simulink model "laguerre"  (R2018b)
settings: Solver=VariableStepAuto  StartTime=0.0  StopTime=5  RelTol=1e-3
undefined symbols (not defined in the file or in its folder): O, p, sigbuilder_block, sigma, Ts
settings Model: Creator=lenovo  LastModifiedBy=lenovo

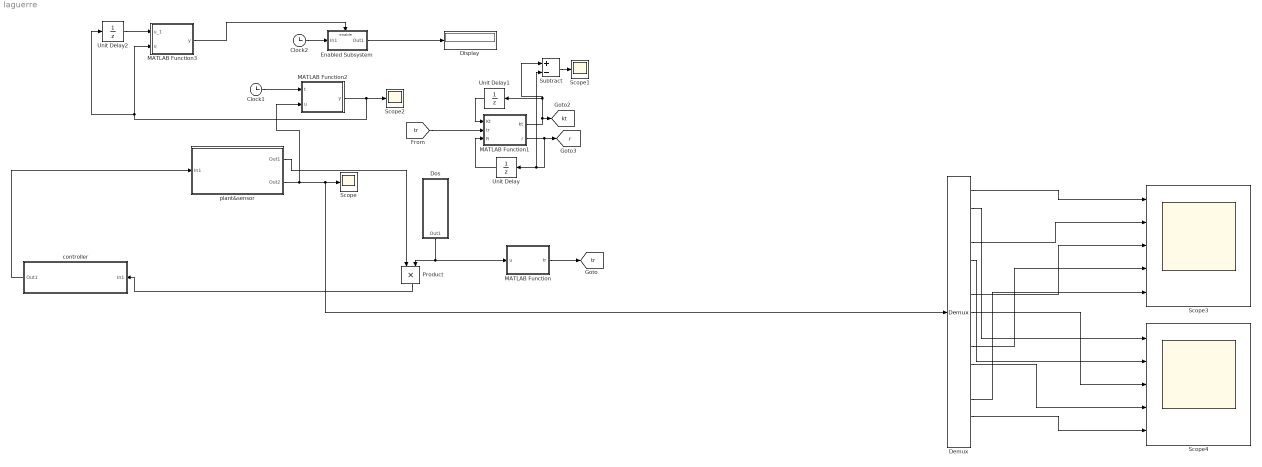
== system laguerre ==
  Clock1 : Clock
  Clock2 : Clock
  Demux : Demux  Outputs=15
  Display : Display
  Dos : Subsystem
  Enabled Subsystem : Subsystem  TreatAsAtomicUnit=on
  MATLAB Function : MATLAB Function  TreatAsAtomicUnit=on
  MATLAB Function1 : MATLAB Function  TreatAsAtomicUnit=on
  MATLAB Function2 : MATLAB Function  TreatAsAtomicUnit=on
  MATLAB Function3 : MATLAB Function  TreatAsAtomicUnit=on
  Product : Product
  Scope : Scope
  Scope1 : Scope
  Scope2 : Scope
  Scope3 : Scope  NumInputPorts=5
  Scope4 : Scope  NumInputPorts=5
  Subtract : Sum  Inputs=+-
  Unit Delay : UnitDelay  SampleTime=0.1
  Unit Delay1 : UnitDelay  SampleTime=0.1
  Unit Delay2 : UnitDelay  SampleTime=0.1
  controller : Subsystem
  "plant&sensor " : Subsystem
  tag scope: kt=global, r=global, tr=global
  wires:
  Dos/1(Out1) -> Product/2, MATLAB Function/1(u)
  controller/1(Out1) -> "plant&sensor "/1(In1)
  Subtract/1 -> Scope1/1
  MATLAB Function2/1(y) -> Unit Delay2/1, MATLAB Function3/2(u), Scope2/1
  MATLAB Function1/2(r) -> Subtract/2, Unit Delay/1, [r]
  "plant&sensor "/1(Out1) -> Product/1
  MATLAB Function1/1(kt) -> Unit Delay1/1, Subtract/1, [kt]
  Product/1 -> controller/1(In1)
  Unit Delay1/1 -> MATLAB Function1/1(Kt)
  [tr] -> MATLAB Function1/2(tr)
  Unit Delay2/1 -> MATLAB Function3/1(u_1)
  Enabled Subsystem/1(Out1) -> Display/1
  Clock1/1 -> MATLAB Function2/1(t)
  MATLAB Function3/1(y) -> Enabled Subsystem/Enable
  Clock2/1 -> Enabled Subsystem/1(In1)
  Unit Delay/1 -> MATLAB Function1/3(R)
  MATLAB Function/1(tr) -> [tr]
  Demux/8 -> Scope4/3
  Demux/11 -> Scope4/4
  Demux/2 -> Scope4/1
  Demux/7 -> Scope3/3
  Demux/4 -> Scope3/2
  Demux/1 -> Scope3/1
  Demux/13 -> Scope3/5
  Demux/10 -> Scope3/4
  "plant&sensor "/2(Out2) -> Demux/1, Scope/1, MATLAB Function2/2(u)
  Demux/14 -> Scope4/5
  Demux/5 -> Scope4/2

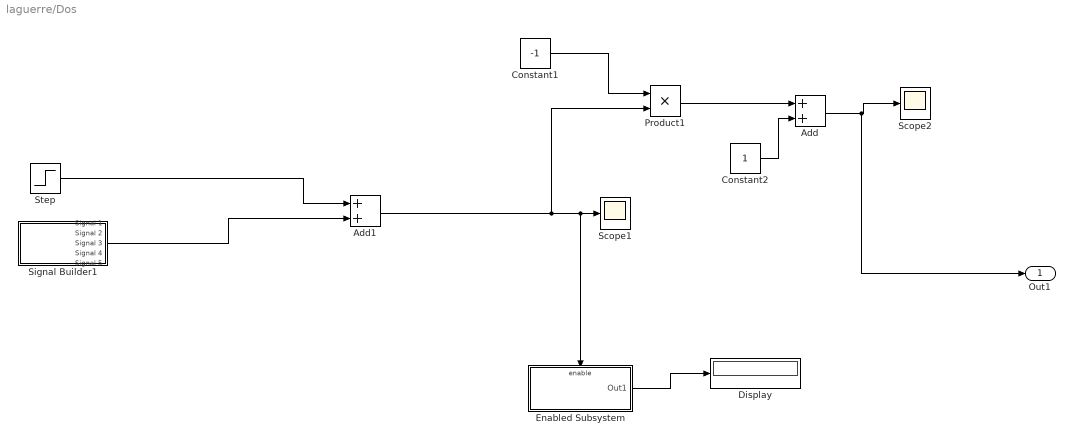
== system laguerre/Dos ==
  Add : Sum
  Add1 : Sum
  Constant1 : Constant  Value=-1
  Constant2 : Constant
  Display : Display
  Enabled Subsystem : Subsystem  TreatAsAtomicUnit=on
  Product1 : Product
  Scope1 : Scope
  Scope2 : Scope
  Signal Builder1 : Subsystem  Tag=STV Subsys  LoadFcn=sigbuilder_block('load');  StartFcn=sigbuilder_block('start');  StopFcn=sigbuilder_block('stop');  ClipboardFcn=sigbuilder_block('clipboard');  mask(Sigbuilder block){tuvar=[0:10]}
      mask help: Simulink:masks:SigbuilderBlock_MD
      mask init:
      | if ~strcmp(get_param(bdroot(gcbh),'SimulationStatus'),'stopped') tuvar = sigbuilder_block('maskInit'); end
      settings: CopyFcn=sigbuilder_block('copy');  DeleteFcn=sigbuilder_block('delete');  ModelCloseFcn=sigbuilder_block('modelClose');  PreSaveFcn=sigbuilder_block('preSave');  PauseFcn=sigbuilder_block('pause');  ContinueFcn=sigbuilder_block('continue');  NameChangeFcn=sigbuilder_block('namechange');  OpenFcn=sigbuilder_block('open',[5.4 30 1141.2 522.6 ]);  CloseFcn=sigbuilder_block('close');
      mask Display: plot(0, 0, 100, 100,[2, 2, 32, 32, 2], [68, 8, 8, 68, 68],[32, 2], [38, 38], [32, 19, 2],[53, 60, 44], [32, 17, 17, 2],[16, 16, 31, 31]);txt = getActiveGroup(gcbh);text(2, 100, txt,'verticalAlignment', 'top');
  Step : Step  After=-1  SampleTime=5
  Out1 : Outport
  wires:
  Enabled Subsystem/1(Out1) -> Display/1
  Constant1/1 -> Product1/1
  Product1/1 -> Add/1
  Constant2/1 -> Add/2
  Add/1 -> Out1/1, Scope2/1
  Signal Builder1/3(Signal 3) -> Add1/2
  Step/1 -> Add1/1
  Add1/1 -> Product1/2, Enabled Subsystem/Enable, Scope1/1

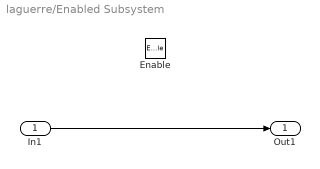
== system laguerre/Enabled Subsystem ==
  In1 : Inport
  Enable : EnablePort
  Out1 : Outport
  wires:
  In1/1 -> Out1/1

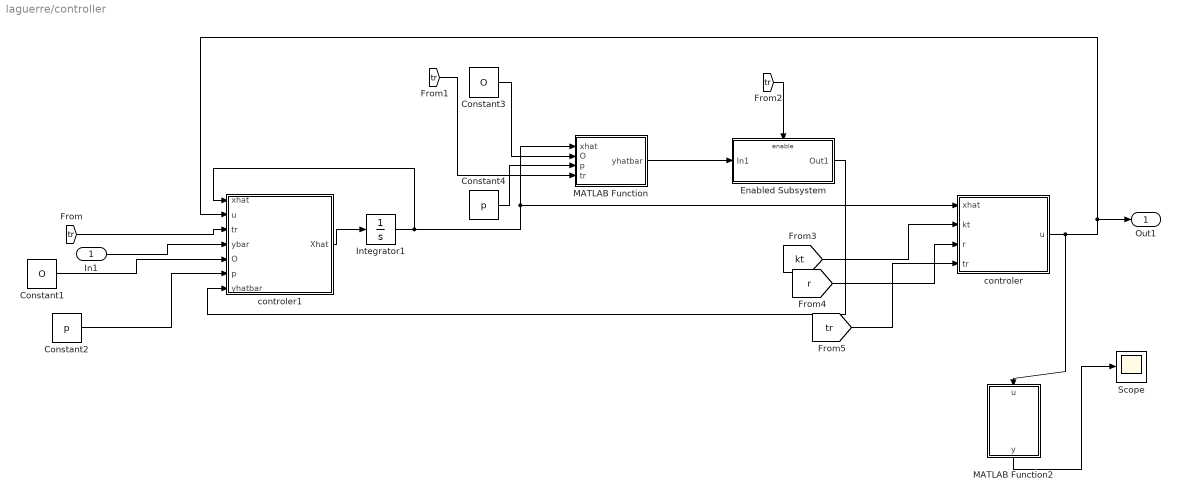
== system laguerre/controller ==
  In1 : Inport
  Constant1 : Constant  Value=O
  Constant2 : Constant  Value=p
  Constant3 : Constant  Value=O
  Constant4 : Constant  Value=p
  Enabled Subsystem : Subsystem  TreatAsAtomicUnit=on
  Integrator1 : Integrator  InitialCondition=[-7;-6;-5;-4;-3;-2;-1;0;1;2;3;4;5;6;7]
  MATLAB Function : MATLAB Function  TreatAsAtomicUnit=on
  MATLAB Function2 : MATLAB Function  TreatAsAtomicUnit=on
  Scope : Scope
  controler : MATLAB Function  TreatAsAtomicUnit=on
  controler1 : MATLAB Function  TreatAsAtomicUnit=on
  Out1 : Outport
  wires:
  controler1/1(Xhat) -> Integrator1/1
  controler/1(u) -> MATLAB Function2/1(u), controler1/2(u), Out1/1
  [tr] -> controler1/3(tr)
  In1/1 -> controler1/4(ybar)
  Constant1/1 -> controler1/5(O)
  Constant3/1 -> MATLAB Function/2(O)
  [tr] -> MATLAB Function/4(tr)
  MATLAB Function/1(yhatbar) -> Enabled Subsystem/1(In1)
  [tr] -> Enabled Subsystem/Enable
  Enabled Subsystem/1(Out1) -> controler1/7(yhatbar)
  [tr] -> controler/4(tr)
  [r] -> controler/3(r)
  [kt] -> controler/2(kt)
  Integrator1/1 -> controler1/1(xhat), controler/1(xhat), MATLAB Function/1(xhat)
  Constant2/1 -> controler1/6(p)
  Constant4/1 -> MATLAB Function/3(p)
  MATLAB Function2/1(y) -> Scope/1

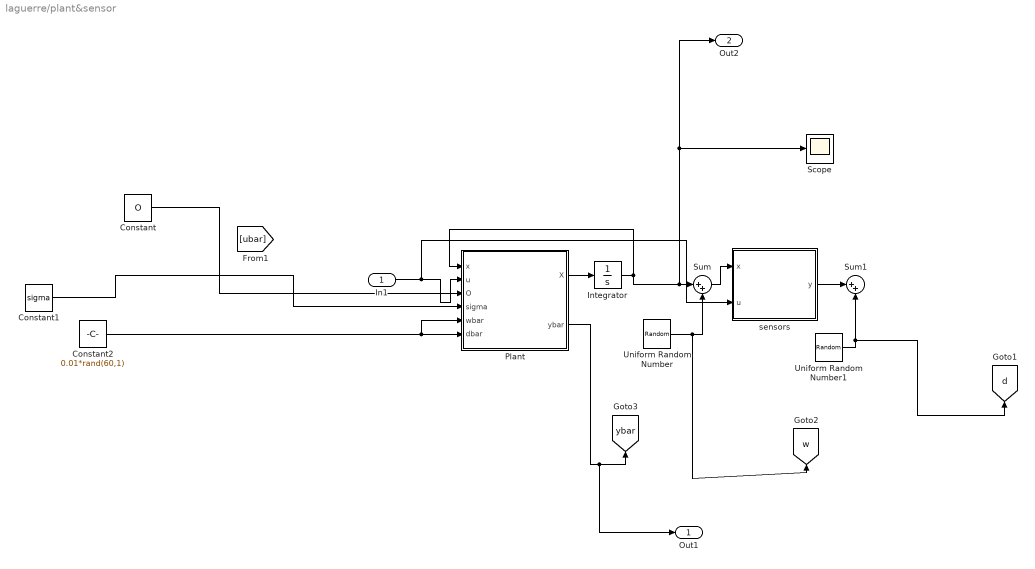
== system laguerre/plant&sensor  ==
  In1 : Inport
  Constant : Constant  Value=O
  Constant1 : Constant  Value=sigma
  Constant2 : Constant  Value=0.01*rand(60,1)
  Integrator : Integrator  InitialCondition=[-7;-6;-5;-4;-3;-2;-1;0;1;2;3;4;5;6;7]
  Plant : MATLAB Function  TreatAsAtomicUnit=on
  Scope : Scope
  Sum : Sum  Inputs=|++
  Sum1 : Sum  Inputs=|++
  Uniform Random Number : UniformRandomNumber  Minimum=-0.01  Maximum=0.01  SampleTime=Ts
  Uniform Random Number1 : UniformRandomNumber  Minimum=-0.01  Maximum=0.01  SampleTime=Ts
  sensors : MATLAB Function  TreatAsAtomicUnit=on
  Out1 : Outport
  Out2 : Outport  Port=2
  tag scope: d=global, w=global, ybar=global
  wires:
  Sum/1 -> sensors/1(x)
  sensors/1(y) -> Sum1/1
  Uniform Random Number1/1 -> [d], Sum1/2
  Plant/1(X) -> Integrator/1
  Integrator/1 -> Out2/1, Scope/1, Sum/1, Plant/1(x)
  Uniform Random Number/1 -> [w], Sum/2
  In1/1 -> sensors/2(u), Plant/2(u)
  Constant/1 -> Plant/3(O)
  Constant1/1 -> Plant/4(sigma)
  Plant/2(ybar) -> Out1/1, [ybar]
  Constant2/1 -> Plant/5(wbar), Plant/6(dbar)

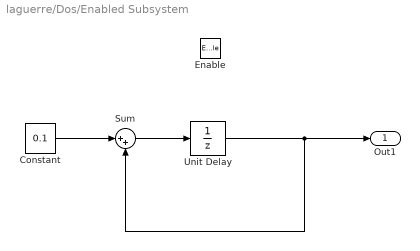
== system laguerre/Dos/Enabled Subsystem ==
  Enable : EnablePort
  Constant : Constant  Value=0.1
  Sum : Sum  Inputs=|++
  Unit Delay : UnitDelay  SampleTime=-1
  Out1 : Outport
  wires:
  Unit Delay/1 -> Out1/1, Sum/2
  Constant/1 -> Sum/1
  Sum/1 -> Unit Delay/1

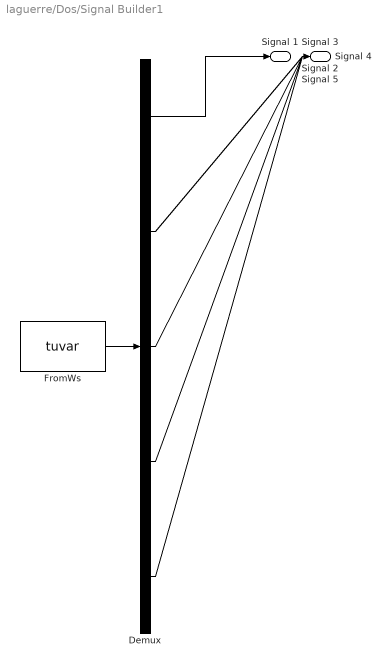
== system laguerre/Dos/Signal Builder1 ==
  Demux : Demux  Tag=STV Demux  Outputs=5
  FromWs : FromWorkspace  Tag=STV FromWs  VariableName=tuvar  SampleTime=0
      SigBuilderData=|
      | common.afterFinalStr = 'Extrapolate'
      | common.sampleTime = 0
      | dataSet.timeRange = [0 10]
      | dataSet.name = 'Group 1'
      | sbobj.Groups.Name = 'Group 1'
      | sbobj.Groups.Signals(1).Name = 'Signal 1'
      | sbobj.Groups.Signals(1).XData = [0 4 4 6 6 10]
      | sbobj.Groups.Signals(1).YData = [0 0 1 1 0 0]
      | sbobj.Groups.Signals(2).Name = 'Signal 2'
      | sbobj.Groups.Signals(2).XData = [0 0.125 0.125 0.25 0.25 0.375 0.375 0.5 0.5 0.625 0.625 0.75 0.75 0.875 0.875 1 1 1.125 1.125 1.25 1.25 1.375 1.375 1.5 1.5 1.625 1.625 1.75 1.75 1.875 1.875 2 2 2.125 2.125 2.25 2.25 2.375 2.375 2.5 2.5 2.625 2.625 2.75 2.75 2.875 2.875 3 3 3.125 3.125 3.25 3.25 3.375 3.375 3.5 3.5 3.625 3.625 3.75 3.75 3.875 3.875 4 4 4.125 4.125 4.25 4.25 4.375 4.375 4.5 4.5 4.625 4.625 4.75 4.75 4.875 4.875 5 5 5.125 5.125 5.25 5.25 5.375 5.375 5.5 5.5 5.625 5.625 5.75 5.75 5.875 5.875 6 6 6.125 6.125 6.25 6.25 6.375 6.375 6.5 6.5 6.625 6.625 6.75 6.75 6.875 6.875 7 7 7.125 7.125 7.25 7.25 7.375 7.375 7.5 7.5 7.625 7.625 7.75 7.75 7.875 7.875 8 8 8.125 8.125 8.25 8.25 8.375 8.375 8.5 8.5 8.625 8.625 8.75 8.75 8.875 8.875 9 9 9.125 9.125 9.25 9.25 9.375 9.375 9.5 9.5 9.625 9.625 9.75 9.75 9.875 9.875 10]
      | sbobj.Groups.Signals(2).YData = [1 1 -1 -1 1 1 -1 -1 1 1 -1 -1 1 1 -1 -1 1 1 -1 -1 1 1 -1 -1 1 1 -1 -1 1 1 -1 -1 1 1 -1 -1 1 1 -1 -1 1 1 -1 -1 1 1 -1 -1 1 1 -1 -1 1 1 -1 -1 1 1 -1 -1 1 1 -1 -1 1 1 -1 -1 1 1 -1 -1 1 1 -1 -1 1 1 -1 -1 1 1 -1 -1 1 1 -1 -1 1 1 -1 -1 1 1 -1 -1 1 1 -1 -1 1 1 -1 -1 1 1 -1 -1 1 1 -1 -1 1 1 -1 -1 1 1 -1 -1 1 1 -1 -1 1 1 -1 -1 1 1 -1 -1 1 1 -1 -1 1 1 -1 -1 1 1 -1 -1 1 1 -1 -1 1 1 -1 -1 1 1 -1 -1 1 1 -1 -1]
      | sbobj.Groups.Signals(3).Name = 'Signal 3'
      | sbobj.Groups.Signals(3).XData = [0 0.16 0.333333333333 0.4 0.4 0.46 0.46 0.833333333333 1 1.005 1.005 1.3 1.3 1.8 1.8 1.9 1.9 2.4 2.4 2.55 2.55 2.625 2.785 2.83333333333 3 3.2 3.2 3.4 3.4 3.5 3.66666666667 3.83333333333 4 4 4.17 4.17 4.33333333333 4.5 4.8 4.8 4.85 4.85 5 5.16666666667 5.33333333333 5.5 5.66666666667 5.83333333333 6 6.16666666667 6.33333333333 6.5 6.66666666667 6.83333333333 7 7.16666666667 7.33333333333 7.5 7.66666666667 7.83333333333 8 8.16666666667 8.33333333333 8.5 8.66666666667 8.83333333333 9 9.16666666667 9.33333333333 9.5 9.66666666667 9.83333333333 10]
      | sbobj.Groups.Signals(3).YData = [1 1 1 1 0 0 1 1 1 1 0 0 1 1 0 0 1 1 0 0 1 1 1 1 1 1 0 0 1 1 1 1 1 0 0 1 1 1 1 0 0 1 1 1 1 1 1 1 1 1 1 1 1 1 1 1 1 1 1 1 1 1 1 1 1 1 1 1 1 1 1 1 1]
      | sbobj.Groups.Signals(4).Name = 'Signal 4'
      | sbobj.Groups.Signals(4).XData = [0 5 5 10]
      | sbobj.Groups.Signals(4).YData = [0 0 1 1]
      | sbobj.Groups.Signals(5).Name = 'Signal 5'
      | sbobj.Groups.Signals(5).XData = [0 0.45 0.45 0.5 0.5 0.95 0.95 1 1 1.45 1.45 1.5 1.5 1.95 1.95 2 2 2.45 2.45 2.5 2.5 2.95 2.95 3 3 3.45 3.45 3.5 3.5 3.95 3.95 4 4 4.45 4.45 4.5 4.5 4.95 4.95 5 5 5.45 5.45 5.5 5.5 5.95 5.95 6 6 6.45 6.45 6.5 6.5 6.95 6.95 7 7 7.45 7.45 7.5 7.5 7.95 7.95 8 8 8.45 8.45 8.5 8.5 8.95 8.95 9 9 9.45 9.45 9.5 9.5 9.95 9.95 10]
      | sbobj.Groups.Signals(5).YData = [2 2 0 0 2 2 0 0 2 2 0 0 2 2 0 0 2 2 0 0 2 2 0 0 2 2 0 0 2 2 0 0 2 2 0 0 2 2 0 0 2 2 0 0 2 2 0 0 2 2 0 0 2 2 0 0 2 2 0 0 2 2 0 0 2 2 0 0 2 2 0 0 2 2 0 0 2 2 0 0]
  Signal 1 : Outport  Tag=STV Outport
  Signal 2 : Outport  Tag=STV Outport  Port=2
  Signal 3 : Outport  Tag=STV Outport  Port=3
  Signal 4 : Outport  Tag=STV Outport  Port=4
  Signal 5 : Outport  Tag=STV Outport  Port=5
  wires:
  Demux/1 -> Signal 1/1
  FromWs/1 -> Demux/1
  Demux/2 -> Signal 2/1
  Demux/3 -> Signal 3/1
  Demux/4 -> Signal 4/1
  Demux/5 -> Signal 5/1

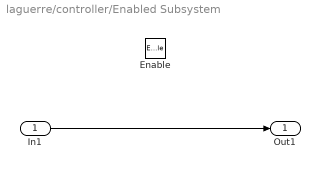
== system laguerre/controller/Enabled Subsystem ==
  In1 : Inport
  Enable : EnablePort
  Out1 : Outport
  wires:
  In1/1 -> Out1/1

== matlab function laguerre/controller/controler ==
  data: xhat input; u output; kt input; r input; tr input
function u = fcn(xhat,kt,r,tr)
K=[1.0766 -.3101 0];
%Kmpc=kron(eye(5),[1 0 0 0])*pinv(F0'*Q*F0+0.1*eye(20))*(F0'*Q*O0)
c=0.1;
L=[ 2 0 0 0 -1; -1 2 0 0 0; -1 0 1 0 0; 0 -1 0 1 0; 0 -1 -1 -1 3];
% u=-c*kron(L,K)*xhat;
K=[1.0766 -.3101 0];
c=0.5;
A=[.9226 -.6330 0;1 0 0;0 1 0];
B=[1;0;0];
L=[ 2 0 0 0 -1; -1 2 0 0 0; -1 0 1 0 0; 0 -1 0 1 0; 0 -1 -1 -1 3];
A0=kron(eye(5),A);
B0=kron(eye(5),B);
z=kron(L,eye(3));
Q=z'*eye(15)*z;
q1=[-0.1356   -0.0988         0   -0.0897   -0.0640         0   -0.0001    0.0008         0
   -0.0283   -0.0192         0    0.0160    0.0151         0    0.0006    0.0015         0
    0.0899    0.0666         0   -0.0847   -0.0553         0    0.0113   -0.0025         0
   -0.0243   -0.0265         0    0.0676    0.0033         0   -0.1854    0.0537         0
    0.0179    0.0060         0   -0.2279    0.0791         0   -0.0045    0.0025         0
];
q2=[0.0021   -0.0002         0    0.0746    0.0555         0
    0.0045    0.0001         0   -0.1103   -0.0802         0
   -0.0067    0.0024         0   -0.1588   -0.1133         0
   -0.2154    0.0521         0    0.1054    0.0639         0
    0.0080   -0.0039         0    0.0028   -0.0071         0
];
q=[q1 q2];
if tr==1
%    u=-c*kron(L,K)*xhat;
u=-c*q*xhat;
else
% u=-c^(kt-r)*kron(eye(5),K*((A-B*K)^(kt-r)))*xhat;
u=-c^(kt-r)*q*((A0-B0*q)^(kt-r))*xhat;
end

== matlab function laguerre/controller/controler1 ==
  data: xhat input; u input; Xhat output; tr input; ybar input; O input; p input; yhatbar input
function Xhat = fcn(xhat,u,tr,ybar,O,p,yhatbar)

  A=[-25.7442 -14.1298 -8.6868;16 0 0;0 16 0];
  B=[8;0;0];
  C=[2.3498 -0.2552 3.3462;3.8307 -3.7641 3.9829;4.4177 -5.2315 4.9];
A_bar=[.9226 -.6330 0;1 0 0;0 1 0];
B_bar=[1;0;0];
C=[2.3498 -0.2552 3.3462;3.8307 -3.7641 3.9829;4.4177 -5.2315 4.9];
G=[0.0450 .0187 .0338;.0005 .0252 .045;-.0631 -.0445 -.0827];
Gsigma=[G,zeros(3,9)];
Fbar=[B_bar zeros(3,3)];
A0=kron(eye(5),A);
B0=kron(eye(5),B);
C0=kron(eye(5),C);
G0=kron(eye(5),G);
Fbar0=kron(eye(5),Fbar);
Gsigma0=kron(eye(5),Gsigma);
O0=kron(eye(5),O);
if tr==1
% FF=[0.4759 0.2743 -.1959 -.0584;0.3476 -.1537 -.0886 .0633;0 0 0 0]';
% FF0=kron(eye(5),FF);
ubar=p*xhat;
Xhat=A0*xhat+Fbar0*ubar+Gsigma0*(ybar-O0*xhat);
else
Xhat=A0*xhat+B0*u+G0*(yhatbar(1:15)-C0*xhat);
end

== matlab function laguerre/controller/MATLAB Function ==
  data: xhat input; yhatbar output; O input; p input; tr input
function yhatbar = fcn(xhat,O,p,tr)
A_bar=[.9226 -.6330 0;1 0 0;0 1 0];
B_bar=[1;0;0];
C_bar=[1 0.2 0.6;0.5 0.6 1.2;0.5 0.9 1.5];
F_bar=[B_bar zeros(3,3)];
FF=[0.4759 0.2743 -.1959 -.0584;0.3476 -.1537 -.0886 .0633;0 0 0 0]';
F=[zeros(3,1) zeros(3,1) zeros(3,1) zeros(3,1);
    C_bar*B_bar zeros(3,1) zeros(3,1) zeros(3,1);
    C_bar*A_bar*B_bar C_bar*B_bar zeros(3,1) zeros(3,1);
    C_bar*A_bar^2*B_bar C_bar*A_bar*B_bar C_bar*B_bar zeros(3,1)];
FF0=kron(eye(5),FF);
F0=kron(eye(5),F);
O0=kron(eye(5),O);
% ubar=FF0*xhat;
ubar=p*xhat;
yhatbar =O0*xhat+F0*ubar;

== matlab function laguerre/MATLAB Function ==
  data: u input; tr output
function tr = fcn(u)
if u==1
    tr=1
else
    tr=0
end

== matlab function laguerre/MATLAB Function3 ==
  data: u_1 input; u input; y output
function y = fcn(u_1,u)
if (u-u_1<.001)
y=0;
else
y=1;
end

== matlab function laguerre/plant&sensor /Plant ==
  data: x input; u input; X output; O input; sigma input; wbar input; dbar input; ybar output
function [X,ybar] = fcn(x,u,O,sigma,wbar,dbar)
A=[-25.7442 -14.1298 -8.6868;16 0 0;0 16 0];
B=[8;0;0];
C=[2.3498 -0.2552 3.3462;3.8307 -3.7641 3.9829;4.4177 -5.2315 4.9];
D=[-.5478;-.4304;-.4304];
A0=kron(eye(5),A);
B0=kron(eye(5),B);
O0=kron(eye(5),O);
sigma0=kron(eye(5),sigma)
X =A0*x+B0*u;
ybar = O0*x+sigma0*wbar+dbar;

== matlab function laguerre/plant&sensor /sensors ==
  data: x input; y output; u input
function y = fcn(x,u)
A=[-25.7442 -14.1298 -8.6868;16 0 0;0 16 0];
B=[8;0;0];
C=[2.3498 -0.2552 3.3462;3.8307 -3.7641 3.9829;4.4177 -5.2315 4.9];
D=[-.5478;-.4304;-.4304];
C0=kron(eye(5),C);
D0=kron(eye(5),D);
y=C0*x+D0*u;

== matlab function laguerre/MATLAB Function2 ==
  data: t input; u input; y output
function y = fcn(t, u)
y=norm(u);

== matlab function laguerre/controller/MATLAB Function2 ==
  data: u input; y output
function y = fcn( u)
y=norm(u);

== matlab function laguerre/MATLAB Function1 ==
  data: kt output; Kt input; tr input; r output; R input
function [kt,r] = fcn( Kt,tr,R)

kt=Kt+1;
if tr==1
    r=R+1
else
    r=R;
end
